simulink model "LQRNonlinearSim"  (R2020a)
settings: Solver=FixedStepAuto  StartTime=0.0  StopTime=5  FixedStep=.01  RelTol=1e-3
values from neighbouring files (symbols this model uses):
  discrete = c2d(continuous, T_s)    [LQR.m]    (also in LQR_Goal_1.m; Naman_LQR_Working.m)
  g = 9.81    [LQR.m]    (also in LQR_Goal_1.m; Naman_LQR_Working.m; PlantModel.m)
  Ix = 4.856*10^-3    (= 0.004856)    [LQR.m]    (also in LQR_Goal_1.m; Naman_LQR_Working.m; PlantModel.m)
  Iy = 4.856*10^-3    (= 0.004856)    [LQR.m]    (also in LQR_Goal_1.m; Naman_LQR_Working.m; PlantModel.m)
  Iz = 8.801*10^-3    (= 0.008801)    [LQR.m]    (also in LQR_Goal_1.m; Naman_LQR_Working.m; PlantModel.m)
  K = zeros(length(R), length(Q), nSteps)    [LQR.m]    (also in LQR_Goal_1.m; Naman_LQR_Working.m)
  m = 0.468    [LQR.m]    (also in LQR_Goal_1.m; Naman_LQR_Working.m; PlantModel.m)
  phi0 = X0(7)    [LQR_Goal_1.m]    (also in PlantModel.m = 0)
  phidot0 = X0(10)    [LQR_Goal_1.m]    (also in PlantModel.m = 0)
  psi0 = X0(9)    [LQR_Goal_1.m]    (also in PlantModel.m = 0)
  psidot0 = X0(12)    [LQR_Goal_1.m]    (also in PlantModel.m = 0)
  theta0 = X0(8)    [LQR_Goal_1.m]    (also in PlantModel.m = 0)
  thetadot0 = X0(11)    [LQR_Goal_1.m]    (also in PlantModel.m = 0)
  x0 = X0(1)    [LQR_Goal_1.m]    (also in PlantModel.m = 0)
  x_0_pitchroll = [0, 0, 0,         0, 0, 0,         10*(pi/180), 10*(pi/180), 0,         0, 0, 0]'    [LQR_Goal_1.m]
  xdot0 = X0(4)    [LQR_Goal_1.m]    (also in PlantModel.m = 0)
  y0 = X0(2)    [LQR_Goal_1.m]    (also in PlantModel.m = 0)
  ydot0 = X0(5)    [LQR_Goal_1.m]    (also in PlantModel.m = 0)
  z0 = X0(3)    [LQR_Goal_1.m]    (also in PlantModel.m = 0)
  zdot0 = X0(6)    [LQR_Goal_1.m]    (also in PlantModel.m = 0)
settings Model: Creator=Lakshu  LastModifiedBy=Lakshu

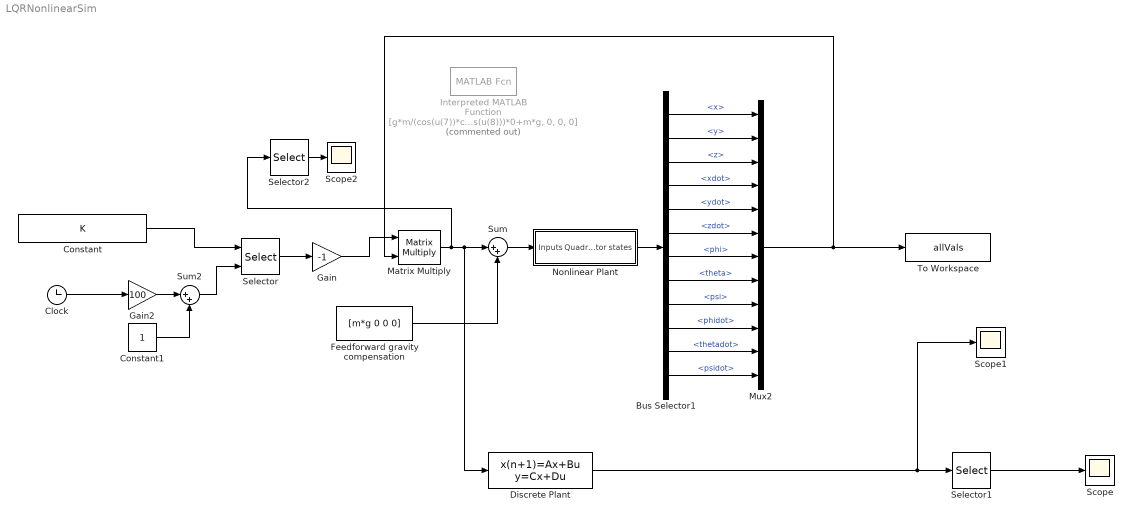
== system LQRNonlinearSim ==
  Bus Selector1 : BusSelector  OutputSignals=x,y,z,xdot,ydot,zdot,phi,theta,psi,phidot,thetadot,psidot
  Clock : Clock
  Constant : Constant  Value=K
  Constant1 : Constant
  Discrete Plant : DiscreteStateSpace  A=discrete.A  B=discrete.B  C=eye(12)  D=zeros(12,4)  InitialCondition=x_0_pitchroll  SampleTime=.01
  Feedforward gravity compensation : Constant  Value=[m*g 0 0 0]
  Gain : Gain  Gain=-1
  Gain2 : Gain  Gain=100
  Interpreted MATLAB Function : MATLABFcn  Commented=on  MATLABFcn=[g*m/(cos(u(7))*cos(u(8)))*0+m*g, 0, 0, 0]  OutputDimensions=4
  Matrix Multiply : Product  Multiplication=Matrix(*)
  Mux2 : Mux  Inputs=12
  Nonlinear Plant : Subsystem
  Scope : Scope
  Scope1 : Scope
  Scope2 : Scope
  Selector : Selector  NumberOfDimensions=3  InputPortWidth=3  IndexOptions=Select all,Select all,Index vector (port)  Indices=[1 3],1,1  OutputSizes=1,1,1
  Selector1 : Selector  InputPortWidth=12  IndexOptions=Index vector (dialog)  Indices=[8]  OutputSizes=1
  Selector2 : Selector  InputPortWidth=4  IndexOptions=Index vector (dialog)  Indices=[1]  OutputSizes=1
  Sum : Sum  Inputs=|++
  Sum2 : Sum  Inputs=|++
  To Workspace : ToWorkspace  VariableName=allVals  SaveFormat=Timeseries  SampleTime=-1
  wires:
  Bus Selector1/2 -> Mux2/2  "<y>"
  Bus Selector1/6 -> Mux2/6  "<zdot>"
  Bus Selector1/12 -> Mux2/12  "<psidot>"
  Selector/1 -> Gain/1
  Bus Selector1/3 -> Mux2/3  "<z>"
  Bus Selector1/11 -> Mux2/11  "<thetadot>"
  Bus Selector1/4 -> Mux2/4  "<xdot>"
  Bus Selector1/5 -> Mux2/5  "<ydot>"
  Bus Selector1/9 -> Mux2/9  "<psi>"
  Gain2/1 -> Sum2/1
  Nonlinear Plant/1(Quadrotor states) -> Bus Selector1/1
  Bus Selector1/1 -> Mux2/1  "<x>"
  Clock/1 -> Gain2/1
  Bus Selector1/10 -> Mux2/10  "<phidot>"
  Constant1/1 -> Sum2/2
  Constant/1 -> Selector/1
  Matrix Multiply/1 -> Selector2/1, Sum/1, Discrete Plant/1
  Sum2/1 -> Selector/2
  Gain/1 -> Matrix Multiply/1
  Selector1/1 -> Scope/1
  Sum/1 -> Nonlinear Plant/1(Inputs)
  Mux2/1 -> Matrix Multiply/2, To Workspace/1
  Discrete Plant/1 -> Scope1/1, Selector1/1
  Bus Selector1/7 -> Mux2/7  "<phi>"
  Bus Selector1/8 -> Mux2/8  "<theta>"
  Selector2/1 -> Scope2/1
  Feedforward gravity compensation/1 -> Sum/2

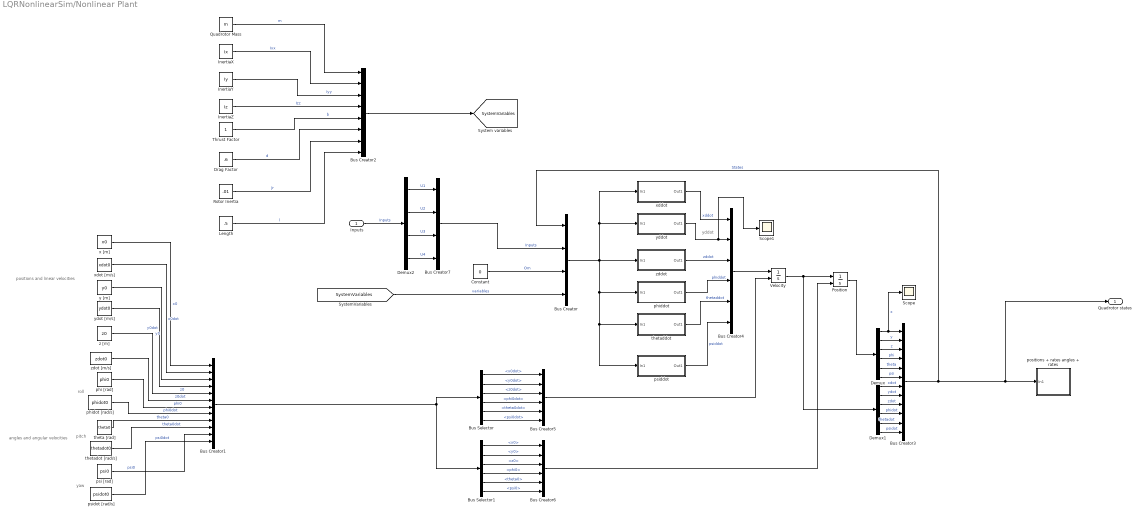
== system LQRNonlinearSim/Nonlinear Plant ==
  note: yddot
  note: positions and linear velocities
  note: pitch
  note: angles and angular velocities
  note: roll
  note: yaw
  Inputs : Inport
  Bus Creator : BusCreator  Inputs=4
  Bus Creator1 : BusCreator  Inputs=12
  Bus Creator2 : BusCreator  Inputs=8
  Bus Creator3 : BusCreator  Inputs=12
  Bus Creator4 : BusCreator  Inputs=6
  Bus Creator5 : BusCreator  Inputs=6
  Bus Creator6 : BusCreator  Inputs=6
  Bus Creator7 : BusCreator  Inputs=4
  Bus Selector : BusSelector  OutputSignals=x0dot,y0dot,z0dot,phi0dot,theta0dot,psi0dot
  Bus Selector1 : BusSelector  OutputSignals=x0,y0,z0,phi0,theta0,psi0
  Constant : Constant  Value=0
  Demux : Demux  Outputs=6
  Demux1 : Demux  Outputs=6
  Demux2 : Demux
  Drag Factor : Constant  Value=.6
  InertiaX : Constant  Value=Ix
  InertiaY : Constant  Value=Iy
  InertiaZ : Constant  Value=Iz
  Length : Constant  Value=.5
  Position : Integrator  InitialConditionSource=external
  Quadrotor Mass : Constant  Value=m
  Rotor Inertia : Constant  Value=.01
  Scope : Scope
  Scope1 : Scope
  Thrust Factor : Constant
  Velocity : Integrator  InitialConditionSource=external
  phi [rad] : Constant  Value=phi0
  phiddot : Subsystem
  phidot [rad/s] : Constant  Value=phidot0
  positions + rates angles + rates : Subsystem
      mask Display: disp('system states')
  psi [rad] : Constant  Value=psi0
  psiddot : Subsystem
  psidot [rad/s] : Constant  Value=psidot0
  theta [rad] : Constant  Value=theta0
  thetaddot : Subsystem
  thetadot [rad/s] : Constant  Value=thetadot0
  x [m] : Constant  Value=x0
  xddot : Subsystem
  xdot [m/s] : Constant  Value=xdot0
  y [m] : Constant  Value=y0
  yddot : Subsystem
  ydot [m/s] : Constant  Value=ydot0
  z [m] : Constant  Value=z0
  zddot : Subsystem
  zdot [m/s] : Constant  Value=zdot0
  Quadrotor states : Outport
  tag scope: SystemVariables=global
  wires:
  [SystemVariables] -> Bus Creator/4  "variables"
  Bus Creator/1 -> xddot/1(In1), yddot/1(In1), zddot/1(In1), phiddot/1(In1), psiddot/1(In1), thetaddot/1(In1)
  xddot/1(Out1) -> Bus Creator4/1  "xddot"
  yddot/1(Out1) -> Scope1/1, Bus Creator4/2
  zddot/1(Out1) -> Bus Creator4/3  "zddot"
  phiddot/1(Out1) -> Bus Creator4/4  "phiddot"
  thetaddot/1(Out1) -> Bus Creator4/5  "thetaddot"
  psiddot/1(Out1) -> Bus Creator4/6  "psiddot"
  Position/1 -> Demux/1
  Bus Creator4/1 -> Velocity/1
  Velocity/1 -> Position/1, Demux1/1
  Bus Creator1/1 -> Bus Selector/1, Bus Selector1/1
  Bus Selector/1 -> Bus Creator5/1  "<x0dot>"
  Bus Selector/2 -> Bus Creator5/2  "<y0dot>"
  Bus Selector/3 -> Bus Creator5/3  "<z0dot>"
  Bus Selector/4 -> Bus Creator5/4  "<phi0dot>"
  Bus Selector/5 -> Bus Creator5/5  "<theta0dot>"
  Bus Selector/6 -> Bus Creator5/6  "<psi0dot>"
  Bus Creator5/1 -> Velocity/2
  Bus Selector1/1 -> Bus Creator6/1  "<x0>"
  Bus Selector1/2 -> Bus Creator6/2  "<y0>"
  Bus Selector1/3 -> Bus Creator6/3  "<z0>"
  Bus Selector1/4 -> Bus Creator6/4  "<phi0>"
  Bus Selector1/5 -> Bus Creator6/5  "<theta0>"
  Bus Selector1/6 -> Bus Creator6/6  "<psi0>"
  Bus Creator6/1 -> Position/2
  Demux/1 -> Scope/1, Bus Creator3/1  "x"
  Demux/2 -> Bus Creator3/2  "y"
  Demux/3 -> Bus Creator3/3  "z"
  Demux/4 -> Bus Creator3/4  "phi"
  Demux/5 -> Bus Creator3/5  "theta"
  Demux/6 -> Bus Creator3/6  "psi"
  Demux1/1 -> Bus Creator3/7  "xdot"
  Demux1/2 -> Bus Creator3/8  "ydot"
  Demux1/3 -> Bus Creator3/9  "zdot"
  Demux1/4 -> Bus Creator3/10  "phidot"
  Demux1/5 -> Bus Creator3/11  "thetadot"
  Demux1/6 -> Bus Creator3/12  "psidot"
  Bus Creator3/1 -> Quadrotor states/1, positions + rates angles + rates/1(In1), Bus Creator/1  "States"
  ydot [m/s]/1 -> Bus Creator1/4  "y0dot"
  psidot [rad/s]/1 -> Bus Creator1/12  "psi0dot"
  x [m]/1 -> Bus Creator1/1  "x0"
  phidot [rad/s]/1 -> Bus Creator1/8  "phi0dot"
  phi [rad]/1 -> Bus Creator1/7  "phi0"
  zdot [m/s]/1 -> Bus Creator1/6  "z0dot"
  y [m]/1 -> Bus Creator1/3  "y0"
  theta [rad]/1 -> Bus Creator1/9  "theta0"
  thetadot [rad/s]/1 -> Bus Creator1/10  "theta0dot"
  z [m]/1 -> Bus Creator1/5  "z0"
  psi [rad]/1 -> Bus Creator1/11  "psi0"
  xdot [m/s]/1 -> Bus Creator1/2  "x0dot"
  Rotor Inertia/1 -> Bus Creator2/7  "Jr"
  Length/1 -> Bus Creator2/8  "l"
  InertiaX/1 -> Bus Creator2/2  "Ixx"
  Drag Factor/1 -> Bus Creator2/6  "d"
  Quadrotor Mass/1 -> Bus Creator2/1  "m"
  Bus Creator2/1 -> [SystemVariables]
  InertiaZ/1 -> Bus Creator2/4  "Izz"
  InertiaY/1 -> Bus Creator2/3  "Iyy"
  Thrust Factor/1 -> Bus Creator2/5  "b"
  Bus Creator7/1 -> Bus Creator/2  "Inputs"
  Constant/1 -> Bus Creator/3  "Om"
  Demux2/1 -> Bus Creator7/1  "U1"
  Demux2/2 -> Bus Creator7/2  "U2"
  Demux2/3 -> Bus Creator7/3  "U3"
  Demux2/4 -> Bus Creator7/4  "U4"
  Inputs/1 -> Demux2/1  "Inputs"

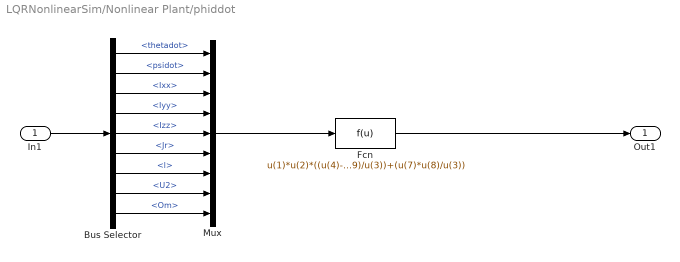
== system LQRNonlinearSim/Nonlinear Plant/phiddot ==
  In1 : Inport
  Bus Selector : BusSelector  OutputSignals=States.thetadot,States.psidot,variables.Ixx,variables.Iyy,variables.Izz,variables.Jr,variables.l,Inputs.U2,Om
  Fcn : Fcn  Expr=u(1)*u(2)*((u(4)-u(5))/u(3))-(u(6)*u(1)*u(9)/u(3))+(u(7)*u(8)/u(3))
  Mux : Mux  Inputs=9
  Out1 : Outport
  wires:
  Bus Selector/7 -> Mux/7  "<l>"
  Mux/1 -> Fcn/1
  Bus Selector/3 -> Mux/3  "<Ixx>"
  Bus Selector/8 -> Mux/8  "<U2>"
  Bus Selector/5 -> Mux/5  "<Izz>"
  Bus Selector/4 -> Mux/4  "<Iyy>"
  Bus Selector/2 -> Mux/2  "<psidot>"
  Bus Selector/1 -> Mux/1  "<thetadot>"
  In1/1 -> Bus Selector/1
  Bus Selector/9 -> Mux/9  "<Om>"
  Fcn/1 -> Out1/1
  Bus Selector/6 -> Mux/6  "<Jr>"

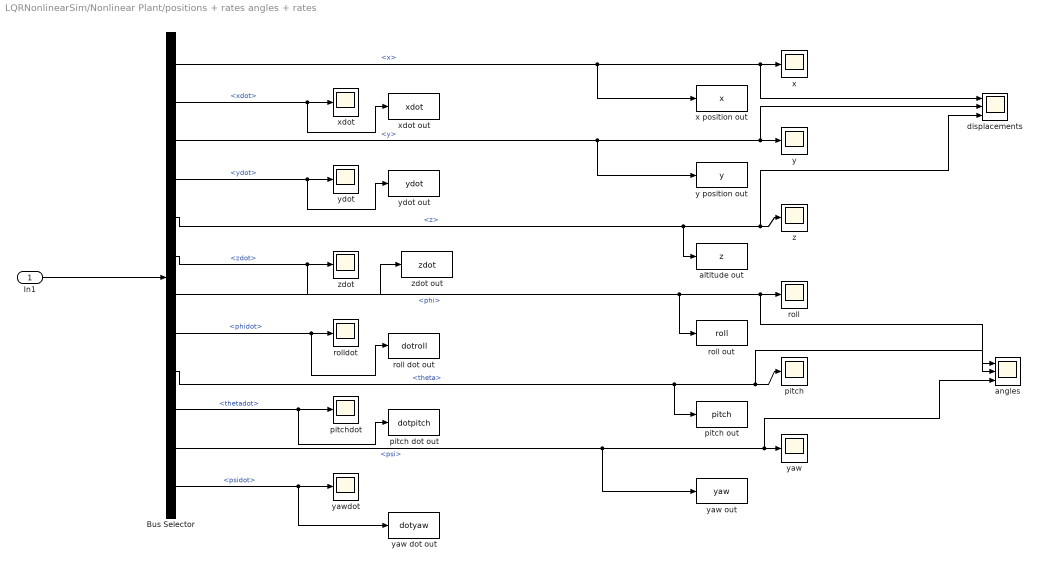
== system LQRNonlinearSim/Nonlinear Plant/positions + rates angles + rates ==
  In1 : Inport
  Bus Selector : BusSelector  OutputSignals=x,xdot,y,ydot,z,zdot,phi,phidot,theta,thetadot,psi,psidot
  altitude out : ToWorkspace  VariableName=z  SampleTime=-1
  angles : Scope  NumInputPorts=3
  displacements : Scope  NumInputPorts=3
  pitch : Scope
  pitch dot out : ToWorkspace  VariableName=dotpitch  SampleTime=-1
  pitch out : ToWorkspace  VariableName=pitch  SampleTime=-1
  pitchdot : Scope
  roll : Scope
  roll dot out : ToWorkspace  VariableName=dotroll  SampleTime=-1
  roll out : ToWorkspace  VariableName=roll  SampleTime=-1
  rolldot : Scope
  x : Scope
  x position out : ToWorkspace  VariableName=x  SampleTime=-1
  xdot : Scope
  xdot out : ToWorkspace  VariableName=xdot  SampleTime=-1
  y : Scope
  y position out : ToWorkspace  VariableName=y  SampleTime=-1
  yaw : Scope
  yaw dot out : ToWorkspace  VariableName=dotyaw  SampleTime=-1
  yaw out : ToWorkspace  VariableName=yaw  SampleTime=-1
  yawdot : Scope
  ydot : Scope
  ydot out : ToWorkspace  VariableName=ydot  SampleTime=-1
  z : Scope
  zdot : Scope
  zdot out : ToWorkspace  VariableName=zdot  SampleTime=-1
  wires:
  Bus Selector/2 -> xdot/1, xdot out/1  "<xdot>"
  Bus Selector/4 -> ydot/1, ydot out/1  "<ydot>"
  Bus Selector/1 -> x position out/1, x/1, displacements/1  "<x>"
  Bus Selector/3 -> y position out/1, y/1, displacements/2  "<y>"
  Bus Selector/12 -> yawdot/1, yaw dot out/1  "<psidot>"
  Bus Selector/11 -> yaw out/1, yaw/1, angles/3  "<psi>"
  In1/1 -> Bus Selector/1
  Bus Selector/10 -> pitchdot/1, pitch dot out/1  "<thetadot>"
  Bus Selector/5 -> altitude out/1, z/1, displacements/3  "<z>"
  Bus Selector/6 -> zdot/1, zdot out/1  "<zdot>"
  Bus Selector/7 -> roll out/1, roll/1, angles/1  "<phi>"
  Bus Selector/8 -> rolldot/1, roll dot out/1  "<phidot>"
  Bus Selector/9 -> pitch out/1, pitch/1, angles/2  "<theta>"

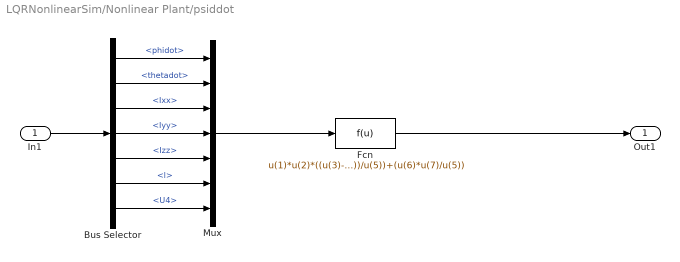
== system LQRNonlinearSim/Nonlinear Plant/psiddot ==
  In1 : Inport
  Bus Selector : BusSelector  OutputSignals=States.phidot,States.thetadot,variables.Ixx,variables.Iyy,variables.Izz,variables.l,Inputs.U4
  Fcn : Fcn  Expr=u(1)*u(2)*((u(3)-u(4))/u(5))+(u(6)*u(7)/u(5))
  Mux : Mux  Inputs=7
  Out1 : Outport
  wires:
  Fcn/1 -> Out1/1
  Mux/1 -> Fcn/1
  In1/1 -> Bus Selector/1
  Bus Selector/1 -> Mux/1  "<phidot>"
  Bus Selector/2 -> Mux/2  "<thetadot>"
  Bus Selector/3 -> Mux/3  "<Ixx>"
  Bus Selector/4 -> Mux/4  "<Iyy>"
  Bus Selector/5 -> Mux/5  "<Izz>"
  Bus Selector/6 -> Mux/6  "<l>"
  Bus Selector/7 -> Mux/7  "<U4>"

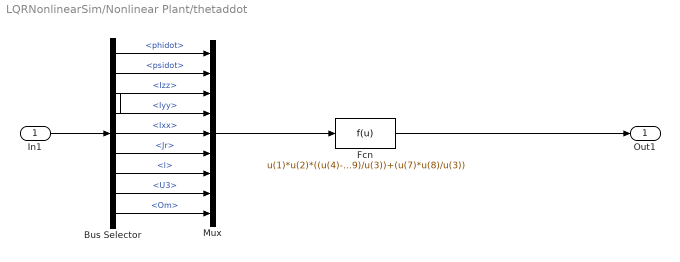
== system LQRNonlinearSim/Nonlinear Plant/thetaddot ==
  In1 : Inport
  Bus Selector : BusSelector  OutputSignals=States.phidot,States.psidot,variables.Iyy,variables.Izz,variables.Ixx,variables.Jr,variables.l,Inputs.U3,Om
  Fcn : Fcn  Expr=u(1)*u(2)*((u(4)-u(5))/u(3))+(u(6)*u(1)*u(9)/u(3))+(u(7)*u(8)/u(3))
  Mux : Mux  Inputs=9
  Out1 : Outport
  wires:
  Bus Selector/1 -> Mux/1  "<phidot>"
  Bus Selector/2 -> Mux/2  "<psidot>"
  Bus Selector/9 -> Mux/9  "<Om>"
  Bus Selector/8 -> Mux/8  "<U3>"
  Bus Selector/7 -> Mux/7  "<l>"
  Bus Selector/6 -> Mux/6  "<Jr>"
  Bus Selector/3 -> Mux/4  "<Iyy>"
  In1/1 -> Bus Selector/1
  Mux/1 -> Fcn/1
  Fcn/1 -> Out1/1
  Bus Selector/4 -> Mux/3  "<Izz>"
  Bus Selector/5 -> Mux/5  "<Ixx>"

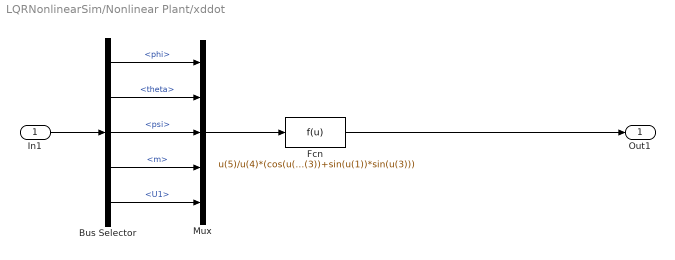
== system LQRNonlinearSim/Nonlinear Plant/xddot ==
  In1 : Inport
  Bus Selector : BusSelector  OutputSignals=States.phi,States.theta,States.psi,variables.m,Inputs.U1
  Fcn : Fcn  Expr=u(5)/u(4)*(cos(u(1))*sin(u(2))*cos(u(3))+sin(u(1))*sin(u(3)))
  Mux : Mux  Inputs=5
  Out1 : Outport
  wires:
  In1/1 -> Bus Selector/1
  Bus Selector/1 -> Mux/1  "<phi>"
  Bus Selector/2 -> Mux/2  "<theta>"
  Bus Selector/3 -> Mux/3  "<psi>"
  Bus Selector/4 -> Mux/4  "<m>"
  Bus Selector/5 -> Mux/5  "<U1>"
  Mux/1 -> Fcn/1
  Fcn/1 -> Out1/1

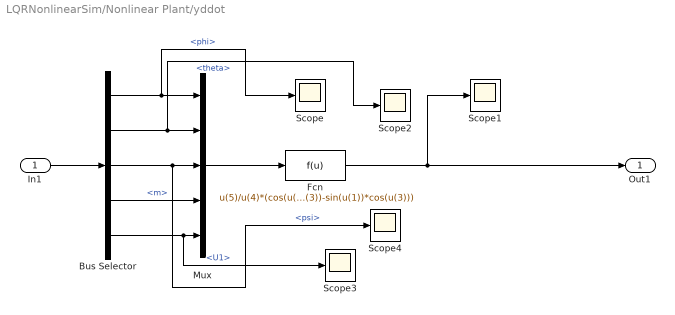
== system LQRNonlinearSim/Nonlinear Plant/yddot ==
  In1 : Inport
  Bus Selector : BusSelector  OutputSignals=States.phi,States.theta,States.psi,variables.m,Inputs.U1
  Fcn : Fcn  Expr=u(5)/u(4)*(cos(u(1))*sin(u(2))*sin(u(3))-sin(u(1))*cos(u(3)))
  Mux : Mux  Inputs=5
  Scope{,1..4} (5 alike) : Scope
  Out1 : Outport
  wires:
  Fcn/1 -> Scope1/1, Out1/1
  Mux/1 -> Fcn/1
  Bus Selector/5 -> Scope3/1, Mux/5  "<U1>"
  Bus Selector/4 -> Mux/4  "<m>"
  Bus Selector/3 -> Scope4/1, Mux/3  "<psi>"
  Bus Selector/2 -> Scope2/1, Mux/2  "<theta>"
  Bus Selector/1 -> Scope/1, Mux/1  "<phi>"
  In1/1 -> Bus Selector/1

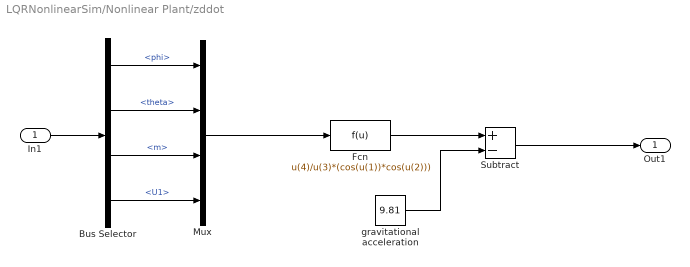
== system LQRNonlinearSim/Nonlinear Plant/zddot ==
  In1 : Inport
  Bus Selector : BusSelector  OutputSignals=States.phi,States.theta,variables.m,Inputs.U1
  Fcn : Fcn  Expr=u(4)/u(3)*(cos(u(1))*cos(u(2)))
  Mux : Mux
  Subtract : Sum  Inputs=+-
  gravitational acceleration : Constant  Value=9.81
  Out1 : Outport
  wires:
  In1/1 -> Bus Selector/1
  Bus Selector/1 -> Mux/1  "<phi>"
  Bus Selector/2 -> Mux/2  "<theta>"
  Mux/1 -> Fcn/1
  Bus Selector/3 -> Mux/3  "<m>"
  Bus Selector/4 -> Mux/4  "<U1>"
  Fcn/1 -> Subtract/1
  gravitational acceleration/1 -> Subtract/2
  Subtract/1 -> Out1/1
